simulink model "Case_Composite_Simulation_InfBus_v1"  (R2020b)
settings: Solver=FixedStepAuto  StartTime=0  StopTime=25  FixedStep=Ts  RelTol=1e-3
undefined symbols (not defined in the file or in its folder): DeviceDiscreDamping, DevicePara, DeviceType, Fbase, OtherInputs, PowerFlow, Sbase, Ts, Vbase, Wbase, x_e, Ybase, Zbase
libraries: powerlib x57, Simplex_PowerSystems x30
settings Model: Creator=admin_user  LastModifiedBy=admin_user
settings DataIOCC: ReturnWorkspaceOutputs=off

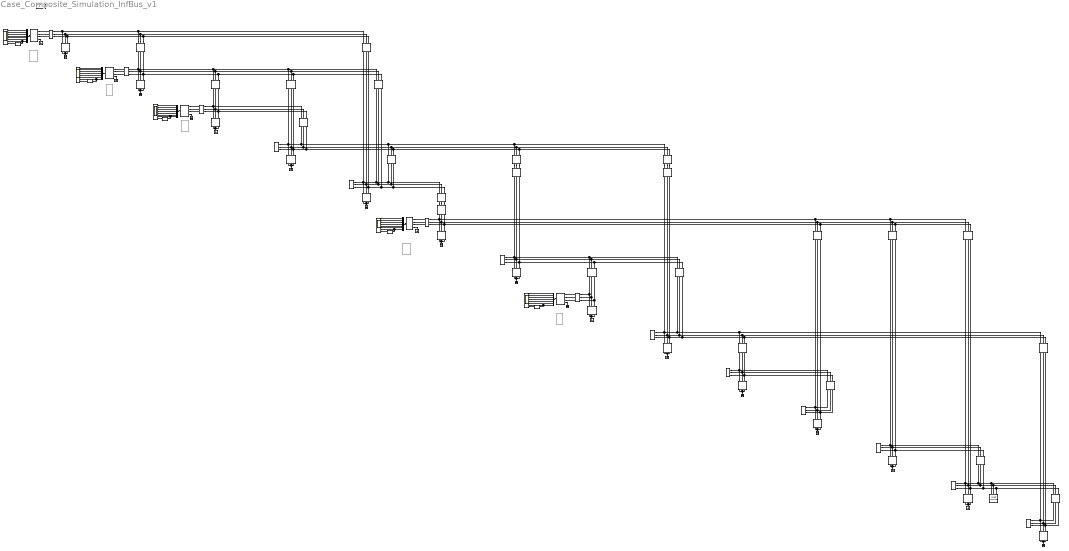
== system Case_Composite_Simulation_InfBus_v1 ==
  B-GND{1,4,8,10,14,16,20,23..24,27,29..30,32,34} (14 alike) : powerlib/Elements/Ground  LConnTagsString=a
  Branch1010 : powerlib/Elements/Three-Phase Parallel RLC Branch  LConnTagsString=A|B|C  RConnTagsString=A|B|C  BranchType=RC  Resistance=(4.7578)*Zbase  Inductance=1e-3  Capacitance=(1e-05)*Ybase/Wbase  Measurements=None
      settings: SourceProductBaseCode=PS
  Branch{12,15,23..25,34,45,78..79,611..613,910,914,1011,1213,1314} (17 alike) : powerlib/Elements/Three-Phase Series RLC Branch  LConnTagsString=A|B|C  RConnTagsString=A|B|C  BranchType=RL  Resistance=(0.01)*Zbase  Inductance=(0.3)*Zbase/Wbase  Capacitance=1e-6  Measurements=None
  Branch11 : powerlib/Elements/Three-Phase Parallel RLC Branch  LConnTagsString=A|B|C  RConnTagsString=A|B|C  BranchType=C  Resistance=(Inf)*Zbase  Inductance=1e-3  Capacitance=(1e-05)*Ybase/Wbase  Measurements=None
      settings: SourceProductBaseCode=PS
  Branch1111 : powerlib/Elements/Three-Phase Parallel RLC Branch  LConnTagsString=A|B|C  RConnTagsString=A|B|C  BranchType=RC  Resistance=(4.959)*Zbase  Inductance=1e-3  Capacitance=(1e-05)*Ybase/Wbase  Measurements=None
      settings: SourceProductBaseCode=PS
  Branch1212 : powerlib/Elements/Three-Phase Parallel RLC Branch  LConnTagsString=A|B|C  RConnTagsString=A|B|C  BranchType=RC  Resistance=(5.0869)*Zbase  Inductance=1e-3  Capacitance=(1e-05)*Ybase/Wbase  Measurements=None
      settings: SourceProductBaseCode=PS
  Branch1313 : powerlib/Elements/Three-Phase Parallel RLC Branch  LConnTagsString=A|B|C  RConnTagsString=A|B|C  BranchType=RC  Resistance=(5.01)*Zbase  Inductance=1e-3  Capacitance=(1e-05)*Ybase/Wbase  Measurements=None
      settings: SourceProductBaseCode=PS
  Branch1414 : powerlib/Elements/Three-Phase Parallel RLC Branch  LConnTagsString=A|B|C  RConnTagsString=A|B|C  BranchType=RC  Resistance=(4.7828)*Zbase  Inductance=1e-3  Capacitance=(1e-05)*Ybase/Wbase  Measurements=None
      settings: SourceProductBaseCode=PS
  Branch22 : powerlib/Elements/Three-Phase Parallel RLC Branch  LConnTagsString=A|B|C  RConnTagsString=A|B|C  BranchType=RC  Resistance=(4.9005)*Zbase  Inductance=1e-3  Capacitance=(1e-05)*Ybase/Wbase  Measurements=None
      settings: SourceProductBaseCode=PS
  Branch33 : powerlib/Elements/Three-Phase Parallel RLC Branch  LConnTagsString=A|B|C  RConnTagsString=A|B|C  BranchType=RC  Resistance=(4.3153)*Zbase  Inductance=1e-3  Capacitance=(1e-05)*Ybase/Wbase  Measurements=None
      settings: SourceProductBaseCode=PS
  Branch44 : powerlib/Elements/Three-Phase Parallel RLC Branch  LConnTagsString=A|B|C  RConnTagsString=A|B|C  BranchType=RC  Resistance=(4.3476)*Zbase  Inductance=1e-3  Capacitance=(1e-05)*Ybase/Wbase  Measurements=None
      settings: SourceProductBaseCode=PS
  Branch47 : powerlib/Elements/Three-Phase Series RLC Branch  LConnTagsString=A|B|C  RConnTagsString=A|B|C  BranchType=RL  Resistance=(0.01)*Zbase  Inductance=(0.03)*Zbase/Wbase  Capacitance=1e-6  Measurements=None
  Branch49 : powerlib/Elements/Three-Phase Series RLC Branch  LConnTagsString=A|B|C  RConnTagsString=A|B|C  BranchType=RL  Resistance=(0.01)*Zbase  Inductance=(0.03)*Zbase/Wbase  Capacitance=1e-6  Measurements=None
  Branch55 : powerlib/Elements/Three-Phase Parallel RLC Branch  LConnTagsString=A|B|C  RConnTagsString=A|B|C  BranchType=RC  Resistance=(4.5852)*Zbase  Inductance=1e-3  Capacitance=(1e-05)*Ybase/Wbase  Measurements=None
      settings: SourceProductBaseCode=PS
  Branch56 : powerlib/Elements/Three-Phase Series RLC Branch  LConnTagsString=A|B|C  RConnTagsString=A|B|C  BranchType=RL  Resistance=(0.01)*Zbase  Inductance=(0.03)*Zbase/Wbase  Capacitance=1e-6  Measurements=None
  Branch66 : powerlib/Elements/Three-Phase Parallel RLC Branch  LConnTagsString=A|B|C  RConnTagsString=A|B|C  BranchType=RC  Resistance=(5.202)*Zbase  Inductance=1e-3  Capacitance=(1e-05)*Ybase/Wbase  Measurements=None
      settings: SourceProductBaseCode=PS
  Branch77 : powerlib/Elements/Three-Phase Parallel RLC Branch  LConnTagsString=A|B|C  RConnTagsString=A|B|C  BranchType=C  Resistance=(Inf)*Zbase  Inductance=1e-3  Capacitance=(1e-05)*Ybase/Wbase  Measurements=None
      settings: SourceProductBaseCode=PS
  Branch88 : powerlib/Elements/Three-Phase Parallel RLC Branch  LConnTagsString=A|B|C  RConnTagsString=A|B|C  BranchType=C  Resistance=(Inf)*Zbase  Inductance=1e-3  Capacitance=(1e-05)*Ybase/Wbase  Measurements=None
      settings: SourceProductBaseCode=PS
  Branch99 : powerlib/Elements/Three-Phase Parallel RLC Branch  LConnTagsString=A|B|C  RConnTagsString=A|B|C  BranchType=RC  Resistance=(4.6002)*Zbase  Inductance=1e-3  Capacitance=(1e-05)*Ybase/Wbase  Measurements=None
      settings: SourceProductBaseCode=PS
  Bus{1..14} (14 alike) : Simplex_PowerSystems/Three-Phase Bus  Vbase=1  Sbase=1
      settings: SourceProductName=Simplex Power Systems
  D-GND{1..3,6,8} (5 alike) : powerlib/Elements/Ground  LConnTagsString=a
  D-Scope{1..3,6,8} (5 alike) : Scope  NumInputPorts=8
  DS-Bus{1..3,6,8} (5 alike) : BusSelector  OutputSignals=v_dq,i_dq,v_abc,i_abc,w,theta,pq
  Digital LPF{,1..4} (5 alike) : Simplex_PowerSystems/Digital LPF  wfil=15*2*pi  Ts=Ts
      settings: SourceProductName=Simplex Power Systems
  Grid-Following_v2 Voltage-Source Inverter (dq-Frame System Object) : Simplex_PowerSystems/Grid-Following_v2 Voltage-Source Inverter (dq-Frame System Object)  Sbase=Sbase  Vbase=Vbase  Wbase=Wbase  DeviceType=DeviceType{3}  DevicePara=DevicePara{3}  PowerFlow=PowerFlow{3}  x0=x_e{3}  OtherInputs=OtherInputs{3}  Ts=Ts  DiscreMethod=Hybrid Trapezoidal  EnableInsideModification=off  DiscreDampingFlag=on  DiscreDampingValue=DeviceDiscreDamping{3}  LinearizationTimes=1  DirectFeedthrough=off
      settings: SourceProductName=Simplex Power Systems
  Grid-Following_v2 Voltage-Source Inverter (dq-Frame System Object)1 : Simplex_PowerSystems/Grid-Following_v2 Voltage-Source Inverter (dq-Frame System Object)  Sbase=Sbase  Vbase=Vbase  Wbase=Wbase  DeviceType=DeviceType{3}  DevicePara=DevicePara{3}  PowerFlow=PowerFlow{3}  x0=x_e{3}  OtherInputs=OtherInputs{3}  Ts=Ts  DiscreMethod=Hybrid Trapezoidal  EnableInsideModification=off  DiscreDampingFlag=on  DiscreDampingValue=DeviceDiscreDamping{3}  LinearizationTimes=1  DirectFeedthrough=off
      settings: SourceProductName=Simplex Power Systems
  Load Impulse : Simplex_PowerSystems/Load Impulse  t0=15  dt=Ts  R=1*2*Zbase
      settings: SourceProductName=Simplex Power Systems
  SM1 : Simplex_PowerSystems/Synchronous Machine (dq-Frame System Object)  Sbase=Sbase  Vbase=Vbase  Wbase=Wbase  DeviceType=DeviceType{1}  DevicePara=DevicePara{1}  PowerFlow=PowerFlow{1}  x0=x_e{1}  OtherInputs=OtherInputs{1}  Ts=Ts  DiscreMethod=Hybrid Trapezoidal  EnableInsideModification=off  DiscreDampingFlag=on  DiscreDampingValue=DeviceDiscreDamping{1}  LinearizationTimes=1  DirectFeedthrough=off
      settings: SourceProductName=Simplex Power Systems
  SM2 : Simplex_PowerSystems/Synchronous Machine (dq-Frame System Object)  Commented=on  Sbase=Sbase  Vbase=Vbase  Wbase=Wbase  DeviceType=DeviceType{2}  DevicePara=DevicePara{2}  PowerFlow=PowerFlow{2}  x0=x_e{2}  OtherInputs=OtherInputs{2}  Ts=Ts  DiscreMethod=Hybrid Trapezoidal  EnableInsideModification=off  DiscreDampingFlag=on  DiscreDampingValue=DeviceDiscreDamping{2}  LinearizationTimes=1  DirectFeedthrough=off
      settings: SourceProductName=Simplex Power Systems
  SM6 : Simplex_PowerSystems/Synchronous Machine (dq-Frame System Object)  Sbase=Sbase  Vbase=Vbase  Wbase=Wbase  DeviceType=DeviceType{6}  DevicePara=DevicePara{6}  PowerFlow=PowerFlow{6}  x0=x_e{6}  OtherInputs=OtherInputs{6}  Ts=Ts  DiscreMethod=Hybrid Trapezoidal  EnableInsideModification=off  DiscreDampingFlag=on  DiscreDampingValue=DeviceDiscreDamping{6}  LinearizationTimes=1  DirectFeedthrough=off
      settings: SourceProductName=Simplex Power Systems
  Synchronous Machine_v2 (dq-Frame System Object) : Simplex_PowerSystems/Synchronous Machine_v2 (dq-Frame System Object)  Sbase=Sbase  Vbase=Vbase  Wbase=Wbase  DeviceType=0  DevicePara=DevicePara{2}  PowerFlow=PowerFlow{2}  x0=x_e{2}  OtherInputs=OtherInputs{2}  Ts=Ts  DiscreMethod=Hybrid Trapezoidal  EnableInsideModification=off  DiscreDampingFlag=on  DiscreDampingValue=DeviceDiscreDamping{2}  LinearizationTimes=1  DirectFeedthrough=off
      settings: SourceProductName=Simplex Power Systems
  Synchronous Machine_v2 (dq-Frame System Object)1 : Simplex_PowerSystems/Synchronous Machine_v2 (dq-Frame System Object)  Commented=on  Sbase=Sbase  Vbase=Vbase  Wbase=Wbase  DeviceType=0  DevicePara=DevicePara{1}  PowerFlow=PowerFlow{1}  x0=x_e{1}  OtherInputs=OtherInputs{1}  Ts=Ts  DiscreMethod=Hybrid Trapezoidal  EnableInsideModification=off  DiscreDampingFlag=on  DiscreDampingValue=DeviceDiscreDamping{1}  LinearizationTimes=1  DirectFeedthrough=off
      settings: SourceProductName=Simplex Power Systems
  Synchronous Machine_v2 (dq-Frame System Object)2 : Simplex_PowerSystems/Synchronous Machine_v2 (dq-Frame System Object)  Commented=on  Sbase=Sbase  Vbase=Vbase  Wbase=Wbase  DeviceType=0  DevicePara=DevicePara{6}  PowerFlow=PowerFlow{6}  x0=x_e{6}  OtherInputs=OtherInputs{6}  Ts=Ts  DiscreMethod=Hybrid Trapezoidal  EnableInsideModification=off  DiscreDampingFlag=on  DiscreDampingValue=DeviceDiscreDamping{6}  LinearizationTimes=1  DirectFeedthrough=off
      settings: SourceProductName=Simplex Power Systems
  Transformer47 : powerlib/Elements/Three-Phase Transformer (Two Windings)  Winding1Connection=Yg  Winding2Connection=Yg  CoreType=Three single-phase transformers  SetSaturation=off  Hysteresis=off  DataFile='hysteresis'  SetInitialFlux=off  Measurements=None  UNITS=pu  NominalPower=[Sbase, Fbase]  Winding1=[0.978*Vbase, 0, 0]  Winding2=[Vbase, 0, 0]  Rm=1e4  Lm=1e4  L0=0.5  Saturation=[ 0,0 ; 0.0024,1.2 ; 1.0,1.52 ]  InitialFluxes=[ 0.8 , -0.8 , 0.7 ]  BreakLoop=off  DiscreteSolver=Trapezoidal iterative  DataType=off  TransfoNumber=1
  Transformer49 : powerlib/Elements/Three-Phase Transformer (Two Windings)  Winding1Connection=Yg  Winding2Connection=Yg  CoreType=Three single-phase transformers  SetSaturation=off  Hysteresis=off  DataFile='hysteresis'  SetInitialFlux=off  Measurements=None  UNITS=pu  NominalPower=[Sbase, Fbase]  Winding1=[0.969*Vbase, 0, 0]  Winding2=[Vbase, 0, 0]  Rm=1e4  Lm=1e4  L0=0.5  Saturation=[ 0,0 ; 0.0024,1.2 ; 1.0,1.52 ]  InitialFluxes=[ 0.8 , -0.8 , 0.7 ]  BreakLoop=off  DiscreteSolver=Trapezoidal iterative  DataType=off  TransfoNumber=1
  Transformer56 : powerlib/Elements/Three-Phase Transformer (Two Windings)  Winding1Connection=Yg  Winding2Connection=Yg  CoreType=Three single-phase transformers  SetSaturation=off  Hysteresis=off  DataFile='hysteresis'  SetInitialFlux=off  Measurements=None  UNITS=pu  NominalPower=[Sbase, Fbase]  Winding1=[0.932*Vbase, 0, 0]  Winding2=[Vbase, 0, 0]  Rm=1e4  Lm=1e4  L0=0.5  Saturation=[ 0,0 ; 0.0024,1.2 ; 1.0,1.52 ]  InitialFluxes=[ 0.8 , -0.8 , 0.7 ]  BreakLoop=off  DiscreteSolver=Trapezoidal iterative  DataType=off  TransfoNumber=1
  VSI-PLL3 : Simplex_PowerSystems/Grid-Following Voltage-Source Inverter (dq-Frame System Object)  Commented=on  Sbase=Sbase  Vbase=Vbase  Wbase=Wbase  DeviceType=DeviceType{3}  DevicePara=DevicePara{3}  PowerFlow=PowerFlow{3}  x0=x_e{3}  OtherInputs=OtherInputs{3}  Ts=Ts  DiscreMethod=Hybrid Trapezoidal  EnableInsideModification=off  DiscreDampingFlag=on  DiscreDampingValue=DeviceDiscreDamping{3}  LinearizationTimes=1  DirectFeedthrough=off
      settings: SourceProductName=Simplex Power Systems
  VSI-PLL8 : Simplex_PowerSystems/Grid-Following Voltage-Source Inverter (dq-Frame System Object)  Commented=on  Sbase=Sbase  Vbase=Vbase  Wbase=Wbase  DeviceType=DeviceType{8}  DevicePara=DevicePara{8}  PowerFlow=PowerFlow{8}  x0=x_e{8}  OtherInputs=OtherInputs{8}  Ts=Ts  DiscreMethod=Hybrid Trapezoidal  EnableInsideModification=off  DiscreDampingFlag=on  DiscreDampingValue=DeviceDiscreDamping{8}  LinearizationTimes=1  DirectFeedthrough=off
      settings: SourceProductName=Simplex Power Systems
  powergui : powerlib/powergui  Priority=1  SimulationMode=Discrete  SampleTime=Ts  frequency=60  Iterations=50  frequencyindice=0  Pbase=100e6  ErrMax=1e-4  UnitsV=kV  UnitsW=MW  buscounter=0  FunctionMessages=off  echomessages=off  EnableUseOfTLC=off  CurrentSourceSwitches=off  DisableSnubberDevices=off  DisableRonSwitches=off  DisableVfSwitches=off  DisplayEquations=off  AutomaticDiscreteSolvers=off  SolverType=Tustin/Backward Euler (TBE)  Interpol=off  ExternalGateDelay=off  methode=off  Ts=100  x0status=blocks  SPID=on  SwTol=0  HookPort=off  NonlinearTolerance=1e-4  nMaxIteration=100  ContinueOnMaxIteration=off  RestoreLinks=warning  ResistiveCurrentMeasurement=off  Frange=[0:2:500]  Ylog=off  Xlog=on  ShowGrid=off  save=off  variable=ZData  structure=0  ZoomFFT=off  StartTime=0.0  cycles=1  DisplayStyle=1  fundamental=60  FreqAxis=off  MaxFrequency=1000  frequencyindicesteady=1  RmsSteady=1  display=off
  wires:
  SM1/1 -> DS-Bus1/1
  DS-Bus1/1 -> D-Scope1/1  "<v_dq>"
  DS-Bus1/2 -> D-Scope1/2  "<i_dq>"
  DS-Bus1/3 -> D-Scope1/3  "<v_abc>"
  DS-Bus1/4 -> D-Scope1/4  "<i_abc>"
  DS-Bus1/5 -> D-Scope1/5  "<w>"
  DS-Bus1/6 -> D-Scope1/6  "<theta>"
  DS-Bus1/7 -> Digital LPF/1, D-Scope1/7  "<pq>"
  Synchronous Machine_v2 (dq-Frame System Object)/1 -> DS-Bus2/1
  DS-Bus2/1 -> D-Scope2/1  "<v_dq>"
  DS-Bus2/2 -> D-Scope2/2  "<i_dq>"
  DS-Bus2/3 -> D-Scope2/3  "<v_abc>"
  DS-Bus2/4 -> D-Scope2/4  "<i_abc>"
  DS-Bus2/5 -> D-Scope2/5  "<w>"
  DS-Bus2/6 -> D-Scope2/6  "<theta>"
  DS-Bus2/7 -> Digital LPF1/1, D-Scope2/7  "<pq>"
  Grid-Following_v2 Voltage-Source Inverter (dq-Frame System Object)/1 -> DS-Bus3/1
  DS-Bus3/1 -> D-Scope3/1  "<v_dq>"
  DS-Bus3/2 -> D-Scope3/2  "<i_dq>"
  DS-Bus3/3 -> D-Scope3/3  "<v_abc>"
  DS-Bus3/4 -> D-Scope3/4  "<i_abc>"
  DS-Bus3/5 -> D-Scope3/5  "<w>"
  DS-Bus3/6 -> D-Scope3/6  "<theta>"
  DS-Bus3/7 -> Digital LPF2/1, D-Scope3/7  "<pq>"
  SM6/1 -> DS-Bus6/1
  DS-Bus6/1 -> D-Scope6/1  "<v_dq>"
  DS-Bus6/2 -> D-Scope6/2  "<i_dq>"
  DS-Bus6/3 -> D-Scope6/3  "<v_abc>"
  DS-Bus6/4 -> D-Scope6/4  "<i_abc>"
  DS-Bus6/5 -> D-Scope6/5  "<w>"
  DS-Bus6/6 -> D-Scope6/6  "<theta>"
  DS-Bus6/7 -> Digital LPF4/1, D-Scope6/7  "<pq>"
  Grid-Following_v2 Voltage-Source Inverter (dq-Frame System Object)1/1 -> DS-Bus8/1
  DS-Bus8/1 -> D-Scope8/1  "<v_dq>"
  DS-Bus8/2 -> D-Scope8/2  "<i_dq>"
  DS-Bus8/3 -> D-Scope8/3  "<v_abc>"
  DS-Bus8/4 -> D-Scope8/4  "<i_abc>"
  DS-Bus8/5 -> D-Scope8/5  "<w>"
  DS-Bus8/6 -> D-Scope8/6  "<theta>"
  DS-Bus8/7 -> Digital LPF3/1, D-Scope8/7  "<pq>"
  Digital LPF/1 -> D-Scope1/8  "pqfil"
  Digital LPF1/1 -> D-Scope2/8  "pqfil"
  Digital LPF2/1 -> D-Scope3/8  "pqfil"
  Digital LPF3/1 -> D-Scope8/8  "pqfil"
  Digital LPF4/1 -> D-Scope6/8  "pqfil"
  connections:
  SM1/LConn1 -- Bus1/LConn1
  SM1/LConn2 -- Bus1/LConn2
  SM1/LConn3 -- Bus1/LConn3
  Synchronous Machine_v2 (dq-Frame System Object)/LConn1 -- Bus2/LConn1
  Synchronous Machine_v2 (dq-Frame System Object)/LConn2 -- Bus2/LConn2
  Synchronous Machine_v2 (dq-Frame System Object)/LConn3 -- Bus2/LConn3
  Grid-Following_v2 Voltage-Source Inverter (dq-Frame System Object)/LConn1 -- Bus3/LConn1
  Grid-Following_v2 Voltage-Source Inverter (dq-Frame System Object)/LConn2 -- Bus3/LConn2
  Grid-Following_v2 Voltage-Source Inverter (dq-Frame System Object)/LConn3 -- Bus3/LConn3
  SM6/LConn1 -- Bus6/LConn1
  SM6/LConn2 -- Bus6/LConn2
  SM6/LConn3 -- Bus6/LConn3
  Grid-Following_v2 Voltage-Source Inverter (dq-Frame System Object)1/LConn1 -- Bus8/LConn1
  Grid-Following_v2 Voltage-Source Inverter (dq-Frame System Object)1/LConn2 -- Bus8/LConn2
  Grid-Following_v2 Voltage-Source Inverter (dq-Frame System Object)1/LConn3 -- Bus8/LConn3
  SM1/LConn4 -- D-GND1/LConn1
  Synchronous Machine_v2 (dq-Frame System Object)/LConn4 -- D-GND2/LConn1
  Grid-Following_v2 Voltage-Source Inverter (dq-Frame System Object)/LConn4 -- D-GND3/LConn1
  SM6/LConn4 -- D-GND6/LConn1
  Grid-Following_v2 Voltage-Source Inverter (dq-Frame System Object)1/LConn4 -- D-GND8/LConn1
  Branch11/RConn1 -- Branch11/RConn2 -- Branch11/RConn3 -- B-GND1/LConn1
  Branch22/RConn1 -- Branch22/RConn2 -- Branch22/RConn3 -- B-GND4/LConn1
  Branch33/RConn1 -- Branch33/RConn2 -- Branch33/RConn3 -- B-GND8/LConn1
  Branch44/RConn1 -- Branch44/RConn2 -- Branch44/RConn3 -- B-GND10/LConn1
  Branch55/RConn1 -- Branch55/RConn2 -- Branch55/RConn3 -- B-GND14/LConn1
  Branch66/RConn1 -- Branch66/RConn2 -- Branch66/RConn3 -- B-GND16/LConn1
  Branch77/RConn1 -- Branch77/RConn2 -- Branch77/RConn3 -- B-GND20/LConn1
  Branch88/RConn1 -- Branch88/RConn2 -- Branch88/RConn3 -- B-GND23/LConn1
  Branch99/RConn1 -- Branch99/RConn2 -- Branch99/RConn3 -- B-GND24/LConn1
  Branch1010/RConn1 -- Branch1010/RConn2 -- Branch1010/RConn3 -- B-GND27/LConn1
  Branch1111/RConn1 -- Branch1111/RConn2 -- Branch1111/RConn3 -- B-GND29/LConn1
  Branch1212/RConn1 -- Branch1212/RConn2 -- Branch1212/RConn3 -- B-GND30/LConn1
  Branch1313/RConn1 -- Branch1313/RConn2 -- Branch1313/RConn3 -- B-GND32/LConn1
  Branch1414/RConn1 -- Branch1414/RConn2 -- Branch1414/RConn3 -- B-GND34/LConn1
  Branch12/RConn1 -- Bus2/RConn1 -- Branch22/LConn1 -- Branch25/LConn1 -- Branch24/LConn1 -- Branch23/LConn1
  Branch12/RConn2 -- Bus2/RConn2 -- Branch22/LConn2 -- Branch25/LConn2 -- Branch24/LConn2 -- Branch23/LConn2
  Branch12/RConn3 -- Bus2/RConn3 -- Branch22/LConn3 -- Branch25/LConn3 -- Branch24/LConn3 -- Branch23/LConn3
  Branch12/LConn1 -- Bus1/RConn1 -- Branch11/LConn1 -- Branch15/LConn1
  Branch12/LConn2 -- Bus1/RConn2 -- Branch11/LConn2 -- Branch15/LConn2
  Branch12/LConn3 -- Bus1/RConn3 -- Branch11/LConn3 -- Branch15/LConn3
  Branch15/RConn1 -- Bus5/RConn1 -- Branch55/LConn1 -- Transformer56/LConn1 -- Branch45/RConn1 -- Branch25/RConn1
  Branch15/RConn2 -- Bus5/RConn2 -- Branch55/LConn2 -- Transformer56/LConn2 -- Branch45/RConn2 -- Branch25/RConn2
  Branch15/RConn3 -- Bus5/RConn3 -- Branch55/LConn3 -- Transformer56/LConn3 -- Branch45/RConn3 -- Branch25/RConn3
  Branch23/RConn1 -- Bus3/RConn1 -- Branch33/LConn1 -- Branch34/LConn1
  Branch23/RConn2 -- Bus3/RConn2 -- Branch33/LConn2 -- Branch34/LConn2
  Branch23/RConn3 -- Bus3/RConn3 -- Branch33/LConn3 -- Branch34/LConn3
  Branch24/RConn1 -- Bus4/RConn1 -- Branch44/LConn1 -- Transformer49/LConn1 -- Transformer47/LConn1 -- Branch45/LConn1 -- Branch34/RConn1
  Branch24/RConn2 -- Bus4/RConn2 -- Branch44/LConn2 -- Transformer49/LConn2 -- Transformer47/LConn2 -- Branch45/LConn2 -- Branch34/RConn2
  Branch24/RConn3 -- Bus4/RConn3 -- Branch44/LConn3 -- Transformer49/LConn3 -- Transformer47/LConn3 -- Branch45/LConn3 -- Branch34/RConn3
  Branch47/RConn1 -- Bus7/RConn1 -- Branch77/LConn1 -- Branch79/LConn1 -- Branch78/LConn1
  Branch47/RConn2 -- Bus7/RConn2 -- Branch77/LConn2 -- Branch79/LConn2 -- Branch78/LConn2
  Branch47/RConn3 -- Bus7/RConn3 -- Branch77/LConn3 -- Branch79/LConn3 -- Branch78/LConn3
  Transformer47/RConn1 -- Branch47/LConn1
  Transformer47/RConn2 -- Branch47/LConn2
  Transformer47/RConn3 -- Branch47/LConn3
  Branch49/RConn1 -- Bus9/RConn1 -- Branch99/LConn1 -- Branch914/LConn1 -- Branch910/LConn1 -- Branch79/RConn1
  Branch49/RConn2 -- Bus9/RConn2 -- Branch99/LConn2 -- Branch914/LConn2 -- Branch910/LConn2 -- Branch79/RConn2
  Branch49/RConn3 -- Bus9/RConn3 -- Branch99/LConn3 -- Branch914/LConn3 -- Branch910/LConn3 -- Branch79/RConn3
  Transformer49/RConn1 -- Branch49/LConn1
  Transformer49/RConn2 -- Branch49/LConn2
  Transformer49/RConn3 -- Branch49/LConn3
  Branch56/RConn1 -- Bus6/RConn1 -- Branch66/LConn1 -- Branch613/LConn1 -- Branch612/LConn1 -- Branch611/LConn1
  Branch56/RConn2 -- Bus6/RConn2 -- Branch66/LConn2 -- Branch613/LConn2 -- Branch612/LConn2 -- Branch611/LConn2
  Branch56/RConn3 -- Bus6/RConn3 -- Branch66/LConn3 -- Branch613/LConn3 -- Branch612/LConn3 -- Branch611/LConn3
  Transformer56/RConn1 -- Branch56/LConn1
  Transformer56/RConn2 -- Branch56/LConn2
  Transformer56/RConn3 -- Branch56/LConn3
  Branch611/RConn1 -- Bus11/RConn1 -- Branch1111/LConn1 -- Branch1011/RConn1
  Branch611/RConn2 -- Bus11/RConn2 -- Branch1111/LConn2 -- Branch1011/RConn2
  Branch611/RConn3 -- Bus11/RConn3 -- Branch1111/LConn3 -- Branch1011/RConn3
  Branch612/RConn1 -- Bus12/RConn1 -- Branch1212/LConn1 -- Branch1213/LConn1
  Branch612/RConn2 -- Bus12/RConn2 -- Branch1212/LConn2 -- Branch1213/LConn2
  Branch612/RConn3 -- Bus12/RConn3 -- Branch1212/LConn3 -- Branch1213/LConn3
  Branch613/RConn1 -- Bus13/RConn1 -- Branch1313/LConn1 -- Load Impulse/LConn1 -- Branch1314/LConn1 -- Branch1213/RConn1
  Branch613/RConn2 -- Bus13/RConn2 -- Branch1313/LConn2 -- Load Impulse/LConn2 -- Branch1314/LConn2 -- Branch1213/RConn2
  Branch613/RConn3 -- Bus13/RConn3 -- Branch1313/LConn3 -- Load Impulse/LConn3 -- Branch1314/LConn3 -- Branch1213/RConn3
  Branch78/RConn1 -- Bus8/RConn1 -- Branch88/LConn1
  Branch78/RConn2 -- Bus8/RConn2 -- Branch88/LConn2
  Branch78/RConn3 -- Bus8/RConn3 -- Branch88/LConn3
  Branch910/RConn1 -- Bus10/RConn1 -- Branch1010/LConn1 -- Branch1011/LConn1
  Branch910/RConn2 -- Bus10/RConn2 -- Branch1010/LConn2 -- Branch1011/LConn2
  Branch910/RConn3 -- Bus10/RConn3 -- Branch1010/LConn3 -- Branch1011/LConn3
  Branch914/RConn1 -- Bus14/RConn1 -- Branch1414/LConn1 -- Branch1314/RConn1
  Branch914/RConn2 -- Bus14/RConn2 -- Branch1414/LConn2 -- Branch1314/RConn2
  Branch914/RConn3 -- Bus14/RConn3 -- Branch1414/LConn3 -- Branch1314/RConn3
